simulink model "LoadFlow116BusNetwork_original"  (R2024a)
settings: Solver=FixedStepDiscrete  StartTime=0.0  StopTime=4.5  FixedStep=75e-6  RelTol=1e-3  EnableMultiTasking=on
undefined symbols (not defined in the file or in its folder): D1, D11, Delta
libraries: spsSeriesRLCBranchLib x164, spsLoadFlowBusLib x116, spsDistributedParametersLineLib x79, spsThreePhaseSeriesRLCLoadLib x60, spsThreePhaseTransformerTwoWindingsLib x52, spsThreePhaseParallelRLCLoadLib x44, spsThreePhaseVIMeasurementLib x44, spsSynchronousMachinepuStandardLib x28, spsExcitationSystemLib x28, spsHydraulicTurbineandGovernorLib x28, spsGenericPowerSystemStabilizerLib x28, spsMultiBandPowerSystemStabilizerLib x28
(part 4 of 15)

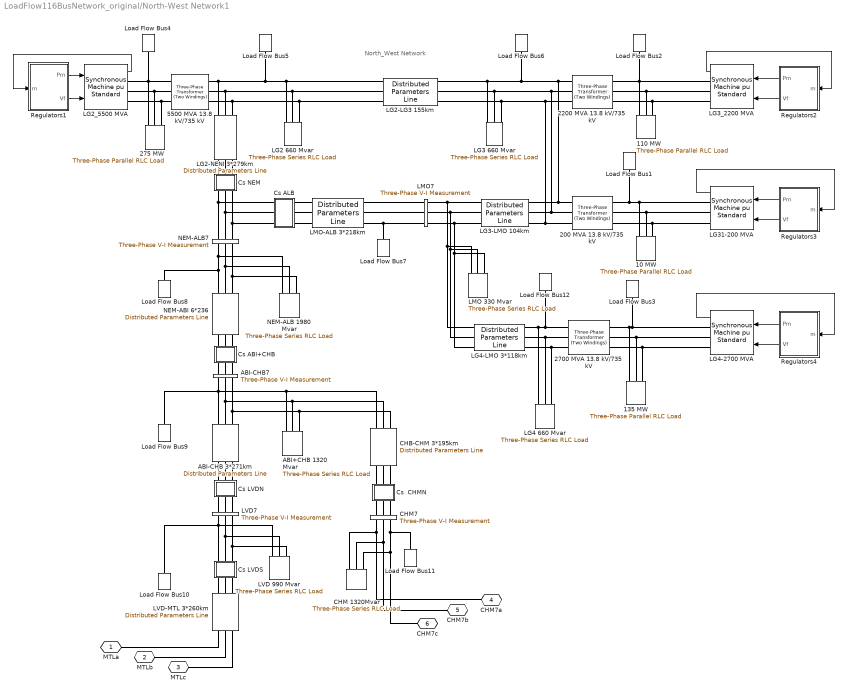
== system LoadFlow116BusNetwork_original/North-West Network1 ==
  note: North_West Network
  10 MW : spsThreePhaseParallelRLCLoadLib/Three-Phase Parallel RLC Load  LConnTagsString=A|B|C  Configuration=Y (grounded)  NominalVoltage=(13800)*1  Vabc=[1e3 1e3 1e3]  Vabcp=[1e3 1e3 1e3]  NominalFrequency=60  UnbalancedPower=off  ActivePower=10000000  InductivePower=0  CapacitivePower=0  Pabc=[10e3 9e3 11e3]  QLabc=[100 90 110]  QCabc=[100 90 110]  Pabcp=[10e3 9e3 11e3]  QLabcp=[100 90 110]  QCabcp=[100 90 110]  Measurements=None  LoadType=constant PQ
  110 MW : spsThreePhaseParallelRLCLoadLib/Three-Phase Parallel RLC Load  LConnTagsString=A|B|C  Configuration=Y (grounded)  NominalVoltage=(13800)*1  Vabc=[1e3 1e3 1e3]  Vabcp=[1e3 1e3 1e3]  NominalFrequency=60  UnbalancedPower=off  ActivePower=110000000  InductivePower=0  CapacitivePower=0  Pabc=[10e3 9e3 11e3]  QLabc=[100 90 110]  QCabc=[100 90 110]  Pabcp=[10e3 9e3 11e3]  QLabcp=[100 90 110]  QCabcp=[100 90 110]  Measurements=None  LoadType=constant PQ
  135 MW : spsThreePhaseParallelRLCLoadLib/Three-Phase Parallel RLC Load  LConnTagsString=A|B|C  Configuration=Y (grounded)  NominalVoltage=(13800)*1  Vabc=[1e3 1e3 1e3]  Vabcp=[1e3 1e3 1e3]  NominalFrequency=60  UnbalancedPower=off  ActivePower=135000000  InductivePower=0  CapacitivePower=0  Pabc=[10e3 9e3 11e3]  QLabc=[100 90 110]  QCabc=[100 90 110]  Pabcp=[10e3 9e3 11e3]  QLabcp=[100 90 110]  QCabcp=[100 90 110]  Measurements=None  LoadType=constant PQ
  200 MVA 13.8 kV/735 kV : spsThreePhaseTransformerTwoWindingsLib/Three-Phase Transformer (Two Windings)  Winding1Connection=Delta (D1)  Winding2Connection=Yg  CoreType=Three single-phase transformers  SetSaturation=off  Hysteresis=off  DataFile='basic_model'  SetInitialFlux=off  Measurements=None  UNITS=pu  NominalPower=[ 200e6 60 ]  Winding1="[ 13.8e3 0.002  0.0]"  Winding2=[ 735e3 0.002 0.12]  Rm=500  Lm=500  L0=0.5  Saturation="[ 0,0  ;  0.005,1.2  ;  1.0,1.4 ]"  InitialFluxes=[ 0.8 , -0.8 , 0.7 ]  BreakLoop=off  DiscreteSolver=Trapezoidal iterative  DataType=off  TransfoNumber=0
  2200 MVA 13.8 kV/735 kV : spsThreePhaseTransformerTwoWindingsLib/Three-Phase Transformer (Two Windings)  Winding1Connection=Delta (D1)  Winding2Connection=Yg  CoreType=Three single-phase transformers  SetSaturation=off  Hysteresis=off  DataFile='basic_model'  SetInitialFlux=off  Measurements=None  UNITS=pu  NominalPower=[ 2200e6 60 ]  Winding1="[ 13.8e3 0.002  0.0]"  Winding2=[ 735e3 0.002 0.12]  Rm=500  Lm=500  L0=0.5  Saturation="[ 0,0  ;  0.005,1.2  ;  1.0,1.4 ]"  InitialFluxes=[ 0.8 , -0.8 , 0.7 ]  BreakLoop=off  DiscreteSolver=Trapezoidal iterative  DataType=off  TransfoNumber=0
  2700 MVA 13.8 kV/735 kV : spsThreePhaseTransformerTwoWindingsLib/Three-Phase Transformer (Two Windings)  Winding1Connection=Delta (D1)  Winding2Connection=Yg  CoreType=Three single-phase transformers  SetSaturation=off  Hysteresis=off  DataFile='basic_model'  SetInitialFlux=off  Measurements=None  UNITS=pu  NominalPower=[ 2700e6 60 ]  Winding1="[ 13.8e3 0.002  0.0]"  Winding2=[ 735e3 0.002 0.12]  Rm=500  Lm=500  L0=0.5  Saturation="[ 0,0  ;  0.005,1.2  ;  1.0,1.4 ]"  InitialFluxes=[ 0.8 , -0.8 , 0.7 ]  BreakLoop=off  DiscreteSolver=Trapezoidal iterative  DataType=off  TransfoNumber=0
  275 MW : spsThreePhaseParallelRLCLoadLib/Three-Phase Parallel RLC Load  LConnTagsString=A|B|C  Configuration=Y (grounded)  NominalVoltage=(13800)*1  Vabc=[1e3 1e3 1e3]  Vabcp=[1e3 1e3 1e3]  NominalFrequency=60  UnbalancedPower=off  ActivePower=275000000  InductivePower=0  CapacitivePower=0  Pabc=[10e3 9e3 11e3]  QLabc=[100 90 110]  QCabc=[100 90 110]  Pabcp=[10e3 9e3 11e3]  QLabcp=[100 90 110]  QCabcp=[100 90 110]  Measurements=None  LoadType=constant PQ
  5500 MVA 13.8 kV/735 kV : spsThreePhaseTransformerTwoWindingsLib/Three-Phase Transformer (Two Windings)  Winding1Connection=Delta (D1)  Winding2Connection=Yg  CoreType=Three single-phase transformers  SetSaturation=off  Hysteresis=off  DataFile='basic_model'  SetInitialFlux=off  Measurements=None  UNITS=pu  NominalPower=[ 5500e6 60 ]  Winding1="[ 13.8e3 0.002  0.0]"  Winding2=[ 735e3 0.002 0.12]  Rm=500  Lm=500  L0=0.5  Saturation="[ 0,0  ;  0.005,1.2  ;  1.0,1.4 ]"  InitialFluxes=[ 0.8 , -0.8 , 0.7 ]  BreakLoop=off  DiscreteSolver=Trapezoidal iterative  DataType=off  TransfoNumber=0
  ABI+CHB 1320 Mvar : spsThreePhaseSeriesRLCLoadLib/Three-Phase Series RLC Load  LConnTagsString=A|B|C  Configuration=Y (grounded)  NominalVoltage=735e3  Vabc=[1e3 1e3 1e3]  Vabcp=[1e3 1e3 1e3]  NominalFrequency=60  UnbalancedPower=off  ActivePower=4400000  InductivePower=1320e6  CapacitivePower=0  Pabc=[10e3 9e3 11e3]  QLabc=[100 90 110]  QCabc=[100 90 110]  Pabcp=[10e3 9e3 11e3]  QLabcp=[100 90 110]  QCabcp=[100 90 110]  Measurements=None  LoadType=constant Z
  ABI-CHB 3*271km : spsDistributedParametersLineLib/Distributed Parameters Line  Phases=3  Length=271  Frequency=60  Resistance="[0.01273  0.3864]/3"  Inductance="[0.9337e-3  4.1264e-3]/3"  Capacitance=[12.74e-9 7.751e-9]*3  x1=[-0.001575 8.53864444420272e-09 -6095.79039975099 -646119.037388367;-0.0015 8.97910610131053e-09 12172.7797949347 -646033.10373521;-0.001425 9.41238999838588e-09 30431.6192557021 -645430.741103565;-0.00135 9.83814977491093e-09 48666.1321456558 -644312.431012903;-0.001275 1.02560450850346e-08 66861.7420741891 -642679.0674232;-0.0012 1.06657418696401e-08 85003.9037491273 -640531.956020319;-0.001125 1.10669126233864e-08 103078.114604012 -637872.813172263;-0.00105 1.14592366565109e-08 121069.92639123 -634703.764557137;-0.000975 1.18424003511844e-08 138964.956731723 -631027.343463919;-0.0009 1.2216097412212e-08 156748.900612039 -626846.488767377;-0.000825 1.25800291118808e-08 174407.541819545 -622164.542578787;-0.00075 1.29339045287585e-08 191926.764306646 -616985.247574297;-0.000675 1.32774407802513e-08 209292.563474937 -611312.744003087;-0.0006 1.36103632487359e-08 226491.057370271 -605151.566377719;-0.000525 1.39324058010851e-08 243508.497779772 -598506.639849319;-0.00045 1.42433110014099e-08 260331.281221952 -591383.276270481;-0.000375 1.45428303168501e-08 276945.959821126 -583787.169949061;-0.0003 1.48307243162478e-08 293339.252057435 -575724.393096226;-0.000225 1.51067628615447e-08 309498.053383889 -567201.390972429;-0.00015 1.53707252917514e-08 325409.446701948 -558224.976735161;-7.5e-05 1.56224005993398e-08 341060.712687245 -548802.325992619]  x2=[-0.001575 1.88534480665931e-08 -248614.692980958 -602078.188381427;-0.0015 1.97916287683191e-08 -231494.235349789 -608866.016701703;-0.001425 2.07139883448297e-08 -214188.724768862 -615167.126844189;-0.00135 2.16197894759921e-08 -196711.994998552 -620976.481797849;-0.001275 2.25083080782413e-08 -179078.016669235 -626289.437653218;-0.0012 2.33788338834014e-08 -161300.886113378 -631101.747314677;-0.001125 2.42306710064632e-08 -143394.814097148 -635409.563895514;-0.00105 2.50631385018642e-08 -125374.114460544 -639209.443793065;-0.000975 2.58755709078257e-08 -107253.192675128 -642498.349441479;-0.0009 2.6667318778313e-08 -89046.5343285159 -645273.651739905;-0.000825 2.74377492021925e-08 -70768.6935448196 -647533.132154148;-0.00075 2.81862463091715e-08 -52434.2813503008 -649274.984490136;-0.000675 2.89122117621149e-08 -34057.953993542 -650497.816337763;-0.0006 2.96150652353474e-08 -15654.401229465 -651200.65018396;-0.000525 3.02942448785564e-08 2761.66542343446 -651382.924194104;-0.00045 3.0949207765927e-08 21175.5244432494 -651044.49266114;-0.000375 3.15794303301483e-08 39572.4560728207 -650185.626122058;-0.0003 3.21844087809452e-08 57937.7540864864 -648807.011141627;-0.000225 3.27636595078005e-08 76256.7375460126 -646909.74976357;-0.00015 3.33167194665461e-08 94514.7625363118 -644495.358629602;-7.5e-05 3.3843146549513e-08 112697.233871564 -641565.767767057]  x3=[-0.001575 -8.90212723717372e-11 -202.312158707681 698.106439471244;-0.0015 -8.43577927577515e-11 -221.966976544963 692.108516415909;-0.001425 -7.96268788149527e-11 -241.444357377404 685.557332402166;-0.00135 -7.48323123635614e-11 -260.72873128478 678.458124346279;-0.001275 -6.99779261066394e-11 -279.804682633651 670.816567246548;-0.0012 -6.5067600566286e-11 -298.656962400379 662.638769646797;-0.001125 -6.01052609816075e-11 -317.270500360969 653.931268753304;-0.00105 -5.50948741709416e-11 -335.630417137972 644.701025209054;-0.000975 -5.00404453608434e-11 -353.722036094833 634.955417529507;-0.0009 -4.49460149843682e-11 -371.530895068167 624.702236204332;-0.000825 -3.98156554512116e-11 -389.042757928598 613.949677469799;-0.00075 -3.46534678922872e-11 -406.243625960894 602.706336756842;-0.000675 -2.94635788813456e-11 -423.119749054334 590.981201819998;-0.0006 -2.42501371362541e-11 -439.657636694328 578.783645552735;-0.000525 -1.90173102025754e-11 -455.844068746536 566.123418494903;-0.00045 -1.37692811220954e-11 -471.666106024837 553.010641038306;-0.000375 -8.51024508896343e-12 -487.111100634715 539.455795336609;-0.0003 -3.24440609611847e-12 -502.166706083795 525.46971692607;-0.000225 2.02402642531864e-12 -516.82088715144 511.063586063777;-0.00015 7.290840971e-12 -531.061929509521 496.248918790319;-7.5e-05 1.25518273299627e-11 -544.878449086672 481.037557724044]  x4=[-0.001575 1.31429208848847e-10 -5039.99478840298 -13897.9312159916;-0.0015 1.32758724317523e-10 -4645.07840312877 -14034.8602322785;-0.001425 1.33982114493257e-10 -4246.44881325117 -14160.5699960362;-0.00135 1.3509840141666e-10 -3844.42467716511 -14274.9600168031;-0.001275 1.36106692745046e-10 -3439.32736681379 -14377.9388529468;-0.0012 1.37006182465753e-10 -3031.48071078892 -14469.4241847613;-0.001125 1.37796151540462e-10 -2621.21073546704 -14549.3428802721;-0.00105 1.38475968479981e-10 -2208.84540438911 -14617.6310536968;-0.000975 1.39045089849051e-10 -1794.71435609138 -14674.2341165144;-0.0009 1.39503060700757e-10 -1379.14864059743 -14719.1068211026;-0.000825 1.39849514940207e-10 -962.480454781879 -14752.213296908;-0.00075 1.40084175617183e-10 -545.042876817216 -14773.5270791201;-0.000675 1.4020685514753e-10 -127.169599916261 -14783.0311298278;-0.0006 1.4021745546311e-10 290.805334417106 -14780.7178516383;-0.000525 1.40115968090191e-10 708.547803415612 -14766.5890937507;-0.00045 1.39902474156227e-10 1125.72387014121 -14740.656150478;-0.000375 1.39577144325002e-10 1542.00005042917 -14702.9397522182;-0.0003 1.39140238660206e-10 1957.04357947021 -14653.470048883;-0.000225 1.38592106417542e-10 2370.5226778176 -14592.2865857963;-0.00015 1.37933185765538e-10 2782.10681660655 -14519.4382720824;-7.5e-05 1.37164003435281e-10 3191.46698177396 -14434.9833415687]  x5=0.00153261764655846  V1=ones(3,3)  V2=ones(3,3)  I1=ones(3,3)  I2=ones(3,3)  nHarmo=1  Measurements=None  Decoupling=off  VsMag0=[ 1 1 1]  VrMag0=[ 1 1 1]  VsAngle0=[0 -120 120]  VrAngle0=[0 -120 120]  IsMag0=[ 1 1 1]  IrMag0=[ 1 1 1]  IsAngle0=[0 -120 120]  IrAngle0=[0 -120 120]
      settings: AttributesFormatString=\n  LibrarySourceBlock=sps_lib/Power Grid Elements/Distributed Parameters Line
  ABI-CHB7 : spsThreePhaseVIMeasurementLib/Three-Phase V-I Measurement  VoltageMeasurement=no  SetLabelV=on  LabelV=Vabc_ABI7  Vpu=on  VpuLL=off  CurrentMeasurement=no  SetLabelI=off  LabelI=A1  Ipu=off  Pbase=100e6  Vbase=500e3  OutputType=Magnitude  PhasorSimulation=off  PSBequivalent=0
  CHB-CHM 3*195km : spsDistributedParametersLineLib/Distributed Parameters Line  Phases=3  Length=195  Frequency=60  Resistance="[0.01273  0.3864]/3"  Inductance="[0.9337e-3  4.1264e-3]/3"  Capacitance=[12.74e-9 7.751e-9]*3  x1=[-0.001125 1.10669126233864e-08 0 0;-0.00105 1.14592366565109e-08 0 0;-0.000975 1.18424003511844e-08 0 0;-0.0009 1.2216097412212e-08 0 0;-0.000825 1.25800291118808e-08 0 0;-0.00075 1.29339045287585e-08 0 0;-0.000675 1.32774407802513e-08 209292.563474937 -611312.744003087;-0.0006 1.36103632487359e-08 226491.057370271 -605151.566377719;-0.000525 1.39324058010851e-08 243508.497779772 -598506.639849319;-0.00045 1.42433110014099e-08 260331.281221952 -591383.276270481;-0.000375 1.45428303168501e-08 276945.959821126 -583787.169949061;-0.0003 1.48307243162478e-08 293339.252057435 -575724.393096226;-0.000225 1.51067628615447e-08 309498.053383889 -567201.390972429;-0.00015 1.53707252917514e-08 325409.446701948 -558224.976735161;-7.5e-05 1.56224005993398e-08 341060.712687245 -548802.325992619]  x2=[-0.001125 8.59552162662043e-09 0 0;-0.00105 8.86565649966125e-09 0 0;-0.000975 9.12870430254534e-09 0 0;-0.0009 9.38445475888383e-09 0 0;-0.000825 9.63270342567504e-09 0 0;-0.00075 9.87325185673308e-09 0 0;-0.000675 1.01059077613227e-08 111004.534524816 -639558.940614591;-0.0006 1.03304851578734e-08 129040.856793898 -636165.151877435;-0.000525 1.05468045226507e-08 146974.025776451 -632262.822451521;-0.00045 1.07546929332641e-08 164789.705971576 -627855.071799286;-0.000375 1.09539842068989e-08 182473.655797114 -622945.423409158;-0.0003 1.11445190331604e-08 200011.738974149 -617537.801978942;-0.000225 1.13261451014236e-08 217389.93582733 -611636.530278469;-0.00015 1.14987172225885e-08 234594.354491989 -605246.325694044;-7.5e-05 1.1662097445142e-08 251611.24201908 -598372.296457439]  x3=[-0.001125 6.30139306376083e-11 0 0;-0.00105 6.39237031354486e-11 0 0;-0.000975 6.47823760030679e-11 0 0;-0.0009 6.55892628305139e-11 0 0;-0.000825 6.63437186048026e-11 0 0;-0.00075 6.70451402255315e-11 0 0;-0.000675 6.76929669869892e-11 49.2476883451471 -2749.35029594662;-0.0006 6.82866810263746e-11 126.95444951433 -2746.85863033986;-0.000525 6.88258077377687e-11 204.55972523904 -2742.17116797236;-0.00045 6.93099161515275e-11 282.001479049262 -2735.2916559298;-0.000375 6.9738619278792e-11 359.2178051919 -2726.22559358886;-0.0003 7.01115744208418e-11 436.146978117284 -2714.98022822106;-0.000225 7.04284834430425e-11 512.727501821634 -2701.5645491994;-0.00015 7.06890930131708e-11 588.898159006021 -2685.98928081244;-7.5e-05 7.08931948039238e-11 664.598060012543 -2668.26687369142]  x4=[-0.001125 -1.1064985641538e-11 0 0;-0.00105 -8.88435086725677e-12 0 0;-0.000975 -6.69661407882735e-12 0 0;-0.0009 -4.50352411956495e-12 0 0;-0.000825 -2.30683411202761e-12 0 0;-0.00075 -1.08300056596849e-13 0 0;-0.000675 2.09032057224212e-12 1717.04187839405 -11467.1483442372;-0.0006 4.2872702307986e-12 2040.53742261431 -11414.0235556945;-0.000525 6.48079271113001e-12 2362.4017924402 -11351.7745713617;-0.00045 8.66913454492761e-12 2682.37769441917 -11280.4511521246;-0.000375 1.08505464052122e-11 3000.20934471098 -11200.1103128332;-0.0003 1.30232845047194e-11 3315.64267355737 -11110.8162767252;-0.000225 1.51856119898564e-11 3628.42552838155 -11012.6404240867;-0.00015 1.73358003291164e-11 3938.30787535512 -10905.6612351922;-7.5e-05 1.947213069484e-11 4245.04199927126 -10789.9642275686]  x5=0.0011028060556417  V1=ones(3,3)  V2=ones(3,3)  I1=ones(3,3)  I2=ones(3,3)  nHarmo=1  Measurements=None  Decoupling=off  VsMag0=[ 1 1 1]  VrMag0=[ 1 1 1]  VsAngle0=[0 -120 120]  VrAngle0=[0 -120 120]  IsMag0=[ 1 1 1]  IrMag0=[ 1 1 1]  IsAngle0=[0 -120 120]  IrAngle0=[0 -120 120]
      settings: AttributesFormatString=\n  LibrarySourceBlock=sps_lib/Power Grid Elements/Distributed Parameters Line
  CHM 1320Mvar : spsThreePhaseSeriesRLCLoadLib/Three-Phase Series RLC Load  LConnTagsString=A|B|C  Configuration=Y (grounded)  NominalVoltage=735e3  Vabc=[1e3 1e3 1e3]  Vabcp=[1e3 1e3 1e3]  NominalFrequency=60  UnbalancedPower=off  ActivePower=4400000  InductivePower=1320e6  CapacitivePower=0  Pabc=[10e3 9e3 11e3]  QLabc=[100 90 110]  QCabc=[100 90 110]  Pabcp=[10e3 9e3 11e3]  QLabcp=[100 90 110]  QCabcp=[100 90 110]  Measurements=None  LoadType=constant Z
  CHM7 : spsThreePhaseVIMeasurementLib/Three-Phase V-I Measurement  VoltageMeasurement=no  SetLabelV=on  LabelV=Vabc_CHM7  Vpu=on  VpuLL=off  CurrentMeasurement=no  SetLabelI=off  LabelI=A1  Ipu=off  Pbase=100e6  Vbase=735e3  OutputType=Magnitude  PhasorSimulation=off  PSBequivalent=0
  "Cs  CHMN " : Subsystem  mask{Xc=25/3}
      mask prompts: Xc "Condensator Reactance at  60Hz  (ohm):"
      mask help: Series Compensation
      mask init:
      | Cs=1/Xc/(2*pi*60);
      mask Display: disp('Cs')
  "Cs ABI+CHB " : Subsystem  mask{Xc=25/6}
      mask prompts: Xc "Condensator Reactance at  60Hz  (ohm):"
      mask help: Series Compensation
      mask init:
      | Cs=1/Xc/(2*pi*60);
      mask Display: disp('Cs')
  Cs ALB : Subsystem  mask{Xc=16/3}
      mask prompts: Xc "Reactance @ 60Hz du condensateur (ohm):"
      mask init:
      | Cs=1/Xc/(2*pi*60);
      mask Display: disp('Cs')
  "Cs LVDN " : Subsystem  mask{Xc=34/3}
      mask prompts: Xc "Condensator Reactance at  60Hz  (ohm):"
      mask help: Series Compensation
      mask init:
      | Cs=1/Xc/(2*pi*60);
      mask Display: disp('Cs')
  "Cs LVDS " : Subsystem  mask{Xc=34/3}
      mask prompts: Xc "Condensator Reactance at  60Hz  (ohm):"
      mask help: Series Compensation
      mask init:
      | Cs=1/Xc/(2*pi*60);
      mask Display: disp('Cs')
  "Cs NEM " : Subsystem  mask{Xc=16/3}
      mask prompts: Xc "Condensator Reactance at  60Hz  (ohm):"
      mask help: Series Compensation
      mask init:
      | Cs=1/Xc/(2*pi*60);
      mask Display: disp('Cs')
  LG2 660 Mvar : spsThreePhaseSeriesRLCLoadLib/Three-Phase Series RLC Load  LConnTagsString=A|B|C  Configuration=Y (grounded)  NominalVoltage=735e3  Vabc=[1e3 1e3 1e3]  Vabcp=[1e3 1e3 1e3]  NominalFrequency=60  UnbalancedPower=off  ActivePower=2200000  InductivePower=660e6  CapacitivePower=0  Pabc=[10e3 9e3 11e3]  QLabc=[100 90 110]  QCabc=[100 90 110]  Pabcp=[10e3 9e3 11e3]  QLabcp=[100 90 110]  QCabcp=[100 90 110]  Measurements=None  LoadType=constant Z
  LG2-LG3 155km : spsDistributedParametersLineLib/Distributed Parameters Line  Phases=3  Length=155  Frequency=60  Resistance="[0.01273  0.3864]"  Inductance="[0.9337e-3  4.1264e-3]"  Capacitance=[12.74e-9 7.751e-9]  x1=[-0.0009 -9.28273050085322e-10 431553.276717529 -473538.091690319;-0.000825 -8.70852358492143e-10 444767.945318795 -461148.506915131;-0.00075 -8.12735520848074e-10 457627.073229751 -448390.287079324;-0.000675 -7.53968994863909e-10 470120.381060296 -435273.630908626;-0.0006 -6.94599757601362e-10 482237.881851304 -421809.023657291;-0.000525 -6.34675267920321e-10 493969.889058048 -408007.228726338;-0.00045 -5.74243428540962e-10 505307.024293471 -393879.279059461;-0.000375 -5.13352547751047e-10 516240.224825131 -379436.468323459;-0.0003 -4.52051300789016e-10 526760.750819806 -364690.341880252;-0.000225 -3.90388690933752e-10 536860.192329986 -349652.687557696;-0.00015 -3.28414010332102e-10 546530.476016653 -334335.526226571;-7.5e-05 -2.66176800595496e-10 555763.871602989 -318751.102191286]  x2=[-0.0009 -4.73016797850604e-10 434484.753049023 -467489.581126984;-0.000825 -4.96742942646812e-10 447527.255751984 -455019.542461771;-0.00075 -5.2007199873509e-10 460212.012014093 -442185.768136346;-0.000675 -5.42985317224948e-10 472528.881835278 -428998.517273542;-0.0006 -5.6546458156017e-10 484468.019298258 -415468.331559927;-0.000525 -5.87491822160791e-10 496019.88043922 -401606.026818942;-0.00045 -6.09049430787703e-10 507175.230877118 -387422.684364896;-0.000375 -6.30120174618412e-10 517925.153195494 -372929.642144734;-0.0003 -6.50687210022693e-10 528261.054070926 -358138.485674657;-0.000225 -6.70734096027131e-10 538174.671142399 -343061.038778834;-0.00015 -6.90244807457779e-10 547658.079616109 -327709.354137622;-7.5e-05 -7.09203747750446e-10 556703.698600424 -312095.703652832]  x3=[-0.0009 8.7944193226646e-12 1522.16056329666 -1950.05893522532;-0.000825 8.80014406364708e-12 1576.68135164224 -1906.24695426432;-0.00075 8.79883410411181e-12 1629.94176503934 -1860.91114865463;-0.000675 8.79049049122039e-12 1681.89922792843 -1814.0877591456;-0.0006 8.7751198947293e-12 1732.51220630862 -1765.81421563838;-0.000525 8.7527346016582e-12 1781.74024093942 -1716.12910726505;-0.00045 8.72335250646786e-12 1829.54397968315 -1665.07215154102;-0.000375 8.68699709675562e-12 1875.88520896249 -1612.68416261551;-0.0003 8.64369743447975e-12 1920.72688430778 -1559.0070186453;-0.000225 8.59348813272776e-12 1964.03315996987 -1504.08362831799;-0.00015 8.53640932804725e-12 2005.76941757459 -1447.95789655146;-7.5e-05 8.47250664836133e-12 2045.90229379621 -1390.67468939692]  x4=[-0.0009 -1.19841358644897e-11 1309.19110331829 -1829.24101140887;-0.000825 -1.1964801318714e-11 1360.38131280582 -1791.49811725853;-0.00075 -1.19359022938317e-11 1410.48405428643 -1752.3231269241;-0.000675 -1.18974618912811e-11 1459.45927639517 -1711.74735629344;-0.0006 -1.18495108397319e-11 1507.26782908884 -1669.80324101677;-0.000525 -1.1792087470521e-11 1553.8714949419 -1626.52431057809;-0.00045 -1.17252376870111e-11 1599.23301969694 -1581.94516149218;-0.000375 -1.16490149278965e-11 1643.31614204512 -1536.10142964875;-0.0003 -1.15634801244843e-11 1686.08562261293 -1489.02976182559;-0.000225 -1.14687016519879e-11 1727.50727213199 -1440.76778639376;-0.00015 -1.13647552748678e-11 1767.54797876946 -1391.35408323796;-7.5e-05 -1.12517240862676e-11 1806.1757345971 -1340.82815291646]  x5=0.000876589428843401  V1=ones(3,3)  V2=ones(3,3)  I1=ones(3,3)  I2=ones(3,3)  nHarmo=1  Measurements=None  Decoupling=off  VsMag0=[ 1 1 1]  VrMag0=[ 1 1 1]  VsAngle0=[0 -120 120]  VrAngle0=[0 -120 120]  IsMag0=[ 1 1 1]  IrMag0=[ 1 1 1]  IsAngle0=[0 -120 120]  IrAngle0=[0 -120 120]
      settings: AttributesFormatString=\n  LibrarySourceBlock=sps_lib/Power Grid Elements/Distributed Parameters Line
  LG2-NENI 3*279km : spsDistributedParametersLineLib/Distributed Parameters Line  Phases=3  Length=279  Frequency=60  Resistance="[0.01273  0.3864]/3"  Inductance="[0.9337e-3  4.1264e-3]/3"  Capacitance=[12.74e-9 7.751e-9]*3  x1=[-0.00165 -1.45441548682992e-09 282305.297313422 -575135.752528875;-0.001575 -1.40637124143826e-09 298451.827359304 -566924.896508615;-0.0015 -1.3572027643944e-09 314359.779580861 -558260.849400328;-0.001425 -1.30694936022658e-09 330016.437404487 -549150.537110708;-0.00135 -1.25565120073718e-09 345409.285137473 -539601.242284006;-0.001275 -1.20334929289003e-09 360526.017972859 -529620.598480399;-0.0012 -1.15008544603e-09 375354.551825711 -519216.584073833;-0.001125 -1.09590223846132e-09 389883.03299295 -508397.515874239;-0.00105 -1.04084298341107e-09 404099.847629026 -497172.042479198;-0.000975 -9.84951694405317e-10 417993.631029841 -485549.137360386;-0.0009 -9.28273050085322e-10 431553.276717529 -473538.091690319;-0.000825 -8.70852358492143e-10 444767.945318795 -461148.506915131;-0.00075 -8.12735520848074e-10 457627.073229751 -448390.287079324;-0.000675 -7.53968994863909e-10 470120.381060296 -435273.630908626;-0.0006 -6.94599757601362e-10 482237.881851304 -421809.023657291;-0.000525 -6.34675267920321e-10 493969.889058048 -408007.228726338;-0.00045 -5.74243428540962e-10 505307.024293471 -393879.279059461;-0.000375 -5.13352547751047e-10 516240.224825131 -379436.468323459;-0.0003 -4.52051300789016e-10 526760.750819806 -364690.341880252;-0.000225 -3.90388690933752e-10 536860.192329986 -349652.687557696;-0.00015 -3.28414010332102e-10 546530.476016653 -334335.526226571;-7.5e-05 -2.66176800595496e-10 555763.871602989 -318751.102191286]  x2=[-0.00165 4.87150453497474e-09 59028.0607460847 -635612.648559132;-0.001575 5.14344828048769e-09 76973.5739080496 -633689.821780515;-0.0015 5.41128043214263e-09 94857.5555727677 -631260.433054146;-0.001425 5.67478688901547e-09 112665.70955893 -628326.424396202;-0.00135 5.93375700807639e-09 130383.800300714 -624890.141208313;-0.001275 6.18798377257458e-09 147997.664227477 -620954.330402681;-0.0012 6.4372639575243e-09 165493.221085897 -616522.138206246;-0.001125 6.68139829215981e-09 182856.485195511 -611597.107645633;-0.00105 6.9201916192294e-09 200073.576628659 -606183.175714918;-0.000975 7.15345305100105e-09 217130.732305878 -600284.67022845;-0.0009 7.38099612185524e-09 234014.316997903 -593906.306361265;-0.000825 7.60263893734264e-09 250710.834225459 -587053.182879846;-0.00075 7.81820431958781e-09 267206.93704814 -579730.778066247;-0.000675 8.02751994892244e-09 283489.438733748 -571944.945338841;-0.0006 8.23041850163507e-09 299545.323299565 -563701.908573182;-0.000525 8.42673778372712e-09 315361.755917135 -555008.257126738;-0.00045 8.61632086056827e-09 330926.093172221 -545870.940571458;-0.000375 8.79901618234761e-09 346225.893171763 -536297.263138391;-0.0003 8.97467770522025e-09 361248.925489739 -526294.877878794;-0.000225 9.14316500805251e-09 375983.180943971 -515871.780546403;-0.00015 9.30434340467244e-09 390416.881196093 -505036.303205745;-7.5e-05 9.45808405153591e-09 404538.488166965 -493797.10757162]  x3=[-0.00165 -4.70582752222005e-11 -180.946605755205 -28.0430826428717;-0.001575 -4.53728751740235e-11 -180.08124143958 -33.1461710872375;-0.0015 -4.36512047436605e-11 -179.071922934883 -38.2227629895896;-0.001425 -4.18946402081113e-11 -177.919457074885 -43.2688002000357;-0.00135 -4.01045857381892e-11 -176.624765123161 -48.2802489936368;-0.001275 -3.82824722760488e-11 -175.188882036646 -53.2531032949049;-0.0012 -3.64297563913123e-11 -173.612955638311 -58.1833878801989;-0.001125 -3.45479191167106e-11 -171.898245699606 -63.0671615554571;-0.00105 -3.26384647641679e-11 -170.04612293342 -67.9005203067278;-0.000975 -3.0702919722278e-11 -168.058067898354 -72.6796004209782;-0.0009 -2.87428312361325e-11 -165.935669815185 -77.4005815746872;-0.000825 -2.67597661704769e-11 -163.680625296466 -82.0596898877539;-0.00075 -2.47553097571828e-11 -161.294736990283 -86.6532009402798;-0.000675 -2.27310643280377e-11 -158.779912139242 -91.1774427498124;-0.0006 -2.06886480338658e-11 -156.138161055851 -95.6287987066725;-0.000525 -1.86296935510025e-11 -153.371595515506 -100.003710465016;-0.00045 -1.65558467761584e-11 -150.48242706837 -104.298680787322;-0.000375 -1.44687655107144e-11 -147.472965271494 -108.51027634003;-0.0003 -1.23701181355006e-11 -144.345615842592 -112.635130438095;-0.000225 -1.02615822771185e-11 -141.102878736948 -116.669945736263;-0.00015 -8.14484346687156e-12 -137.747346148987 -120.611496864919;-7.5e-05 -6.02159379337746e-12 -134.28170044012 -124.456633008399]  x4=[-0.00165 4.85330925004575e-11 1481.48089108514 -13945.3845775473;-0.001575 4.8116399182976e-11 1875.13150496029 -13897.9289700678;-0.0015 4.76612423521933e-11 2267.28316740084 -13839.3635708151;-0.001425 4.71679858535157e-11 2657.62239836797 -13769.7351960732;-0.00135 4.66370239886411e-11 3045.83716665283 -13689.0995056996;-0.001275 4.60687812003605e-11 3431.61713930954 -13597.5209586313;-0.0012 4.54637117332642e-11 3814.65392973059 -13495.0727613578;-0.001125 4.48222992706266e-11 4194.64134416638 -13381.8368094004;-0.00105 4.41450565477561e-11 4571.2756264918 -13257.9036218466;-0.000975 4.34325249421234e-11 4944.25570102427 -13123.3722689901;-0.0009 4.26852740405918e-11 5313.28341319899 -12978.3502931362;-0.000825 4.19039011840989e-11 5678.06376790915 -12822.9536226333;-0.00075 4.10890309901505e-11 6038.30516532055 -12657.3064792023;-0.000675 4.02413148535119e-11 6393.71963397195 -12481.5412786351;-0.0006 3.93614304254921e-11 6744.02306097514 -12295.7985249437;-0.000525 3.84500810722403e-11 7088.93541913041 -12100.2266980435;-0.00045 3.75079953124852e-11 7428.18099077597 -11894.9821350606;-0.000375 3.6535926235169e-11 7761.48858819248 -11680.2289053583;-0.0003 3.55346508974388e-11 8088.59177038635 -11456.1386793825;-0.000225 3.45049697034795e-11 8409.22905607858 -11222.8905914312;-0.00015 3.34477057646831e-11 8723.1441327289 -10980.671096457;-7.5e-05 3.23637042416654e-11 9030.0860614281 -10729.6738210183]  x5=0.00157786097191812  V1=ones(3,3)  V2=ones(3,3)  I1=ones(3,3)  I2=ones(3,3)  nHarmo=1  Measurements=None  Decoupling=off  VsMag0=[ 1 1 1]  VrMag0=[ 1 1 1]  VsAngle0=[0 -120 120]  VrAngle0=[0 -120 120]  IsMag0=[ 1 1 1]  IrMag0=[ 1 1 1]  IsAngle0=[0 -120 120]  IrAngle0=[0 -120 120]
      settings: AttributesFormatString=\n  LibrarySourceBlock=sps_lib/Power Grid Elements/Distributed Parameters Line
  LG2_5500 MVA : spsSynchronousMachinepuStandardLib/Synchronous Machine pu Standard  PresetModel=No  MechanicalLoad=Mechanical power Pm  ShowDetailedParameters=on  RotorType=Salient-pole  Units=per unit standard parameters  MeasurementBus=off  NominalParameters="[5500E6  13800   60 ]"  Reactances1=[ 31 32 33 34 35 36 37 ]  Reactances2=[ 1.305, 0.296, 0.252, 0.474, 0.243, 0.18 ]  dAxisTimeConstants=Short-circuit  qAxisTimeConstants=Open-circuit  TimeConstants1=[]  TimeConstants2=[]  TimeConstants3=[]  TimeConstants4=[]  TimeConstants5=[ 1.01, 0.053, 0.1 ]  TimeConstants6=[]  TimeConstants7=[]  TimeConstants8=[]  StatorResistance=2.8544e-3  Mechanical="[ 4.1  0  32]"  PolePairs=32  InitialConditions=[0 -65.2434 0.985682 0.985682 0.985682 -1.22427 -121.224 118.776 1.47412]  SetSaturation=off  Saturation=[0.6404,0.7127,0.8441,0.9214,0.9956,1.082,1.19,1.316,1.457;0.7,0.7698,0.8872,0.9466,0.9969,1.046,1.1,1.151,1.201]  LoadFlowParameters=[2 4000000000 0 0 0]  TsPowergui=0  TsBlock=-1  IterativeModel=Trapezoidal non iterative  IterativeDiscreteModel=Trapezoidal non iterative  BusType=swing  Pref=0  Qref=0  Qmin=-Inf  Qmax=Inf  PLF=0  QLF=0
  LG3 660 Mvar : spsThreePhaseSeriesRLCLoadLib/Three-Phase Series RLC Load  LConnTagsString=A|B|C  Configuration=Y (grounded)  NominalVoltage=735e3  Vabc=[1e3 1e3 1e3]  Vabcp=[1e3 1e3 1e3]  NominalFrequency=60  UnbalancedPower=off  ActivePower=2200000  InductivePower=660e6  CapacitivePower=0  Pabc=[10e3 9e3 11e3]  QLabc=[100 90 110]  QCabc=[100 90 110]  Pabcp=[10e3 9e3 11e3]  QLabcp=[100 90 110]  QCabcp=[100 90 110]  Measurements=None  LoadType=constant Z
  LG3-LMO 104km : spsDistributedParametersLineLib/Distributed Parameters Line  Phases=3  Length=104  Frequency=60  Resistance="[0.01273  0.3864]"  Inductance="[0.9337e-3  4.1264e-3]"  Capacitance=[12.74e-9 7.751e-9]  x1=[-0.0006 -5.6546458156017e-10 0 0;-0.000525 -5.87491822160791e-10 0 0;-0.00045 -6.09049430787703e-10 0 0;-0.000375 -6.30120174618412e-10 517925.153195494 -372929.642144734;-0.0003 -6.50687210022693e-10 528261.054070926 -358138.485674657;-0.000225 -6.70734096027131e-10 538174.671142399 -343061.038778834;-0.00015 -6.90244807457779e-10 547658.079616109 -327709.354137622;-7.5e-05 -7.09203747750446e-10 556703.698600424 -312095.703652832]  x2=[-0.0006 2.62559334955073e-09 0 0;-0.000525 2.68721757878452e-09 0 0;-0.00045 2.74669368740163e-09 0 0;-0.000375 2.80397413111085e-09 463443.99687782 -442193.458727678;-0.0003 2.85901312080191e-09 475759.806920902 -428914.853919972;-0.000225 2.91176665914857e-09 487695.3018537 -415293.38114066;-0.00015 2.96219257577943e-09 499240.940624185 -401339.929186666;-7.5e-05 3.01025056098827e-09 510387.493825377 -387065.652233986]  x3=[-0.0006 -1.23301013005406e-11 0 0;-0.000525 -1.17759417137608e-11 0 0;-0.00045 -1.12123686193529e-11 0 0;-0.000375 -1.06398325290256e-11 -131.246118914422 -82.6228309096625;-0.0003 -1.00587911193696e-11 -128.857332347406 -86.2998428111622;-0.000225 -9.46970886599742e-12 -126.365539200496 -89.9078679387506;-0.00015 -8.87305667224916e-12 -123.772731375006 -93.4440220923452;-7.5e-05 -8.26931149275942e-12 -121.080981521842 -96.9054785244207]  x4=[-0.0006 1.46115216100586e-11 0 0;-0.000525 1.40654778018821e-11 0 0;-0.00045 1.35081902659598e-11 0 0;-0.000375 1.29401044894211e-11 3539.61351587974 -3162.16565183065;-0.0003 1.23616745913438e-11 3627.594285019 -3060.83488284546;-0.000225 1.17733629597382e-11 3712.67521079086 -2957.05732928728;-0.00015 1.11756398819211e-11 3794.78828080505 -2850.91594934455;-7.5e-05 1.05689831685753e-11 3873.86785512978 -2742.49559081239]  x5=0.000588163229675572  V1=ones(3,3)  V2=ones(3,3)  I1=ones(3,3)  I2=ones(3,3)  nHarmo=1  Measurements=None  Decoupling=off  VsMag0=[ 1 1 1]  VrMag0=[ 1 1 1]  VsAngle0=[0 -120 120]  VrAngle0=[0 -120 120]  IsMag0=[ 1 1 1]  IrMag0=[ 1 1 1]  IsAngle0=[0 -120 120]  IrAngle0=[0 -120 120]
      settings: AttributesFormatString=\n  LibrarySourceBlock=sps_lib/Power Grid Elements/Distributed Parameters Line
  LG31-200 MVA : spsSynchronousMachinepuStandardLib/Synchronous Machine pu Standard  PresetModel=No  MechanicalLoad=Mechanical power Pm  ShowDetailedParameters=on  RotorType=Salient-pole  Units=per unit standard parameters  MeasurementBus=off  NominalParameters="[200E6  13800   60 ]"  Reactances1=[ 31 32 33 34 35 36 37 ]  Reactances2=[ 1.305, 0.296, 0.252, 0.474, 0.243, 0.18 ]  dAxisTimeConstants=Short-circuit  qAxisTimeConstants=Open-circuit  TimeConstants1=[]  TimeConstants2=[]  TimeConstants3=[]  TimeConstants4=[]  TimeConstants5=[ 1.01, 0.053, 0.1 ]  TimeConstants6=[]  TimeConstants7=[]  TimeConstants8=[]  StatorResistance=2.8544e-3  Mechanical="[ 3.2  0  32]"  PolePairs=32  InitialConditions=[0 -67.6291 0.902477 0.902477 0.902477 -4.2812 -124.281 115.719 1.45511]  SetSaturation=off  Saturation=[0.6404,0.7127,0.8441,0.9214,0.9956,1.082,1.19,1.316,1.457;0.7,0.7698,0.8872,0.9466,0.9969,1.046,1.1,1.151,1.201]  LoadFlowParameters=[1 180000000 0 0 0]  TsPowergui=0  TsBlock=-1  IterativeModel=Trapezoidal non iterative  IterativeDiscreteModel=Trapezoidal non iterative  BusType=PV  Pref=180000000  Qref=0  Qmin=-Inf  Qmax=Inf  PLF=0  QLF=0
  LG3_2200 MVA : spsSynchronousMachinepuStandardLib/Synchronous Machine pu Standard  PresetModel=No  MechanicalLoad=Mechanical power Pm  ShowDetailedParameters=on  RotorType=Salient-pole  Units=per unit standard parameters  MeasurementBus=off  NominalParameters="[2200E6  13800   60 ]"  Reactances1=[ 31 32 33 34 35 36 37 ]  Reactances2=[ 1.305, 0.296, 0.252, 0.474, 0.243, 0.18 ]  dAxisTimeConstants=Short-circuit  qAxisTimeConstants=Open-circuit  TimeConstants1=[]  TimeConstants2=[]  TimeConstants3=[]  TimeConstants4=[]  TimeConstants5=[ 1.01, 0.053, 0.1 ]  TimeConstants6=[]  TimeConstants7=[]  TimeConstants8=[]  StatorResistance=2.8544e-3  Mechanical="[ 3.2  0  32]"  PolePairs=32  InitialConditions=[0 -70.0065 0.820496 0.820496 0.820496 -4.90643 -124.906 115.094 1.38903]  SetSaturation=off  Saturation=[0.6404,0.7127,0.8441,0.9214,0.9956,1.082,1.19,1.316,1.457;0.7,0.7698,0.8872,0.9466,0.9969,1.046,1.1,1.151,1.201]  LoadFlowParameters=[1 1800000000 0 0 0]  TsPowergui=0  TsBlock=-1  IterativeModel=Trapezoidal non iterative  IterativeDiscreteModel=Trapezoidal non iterative  BusType=PV  Pref=1800000000  Qref=0  Qmin=-Inf  Qmax=Inf  PLF=0  QLF=0
  LG4 660 Mvar : spsThreePhaseSeriesRLCLoadLib/Three-Phase Series RLC Load  LConnTagsString=A|B|C  Configuration=Y (grounded)  NominalVoltage=735e3  Vabc=[1e3 1e3 1e3]  Vabcp=[1e3 1e3 1e3]  NominalFrequency=60  UnbalancedPower=off  ActivePower=2200000  InductivePower=660e6  CapacitivePower=0  Pabc=[10e3 9e3 11e3]  QLabc=[100 90 110]  QCabc=[100 90 110]  Pabcp=[10e3 9e3 11e3]  QLabcp=[100 90 110]  QCabcp=[100 90 110]  Measurements=None  LoadType=constant Z
  LG4-2700 MVA : spsSynchronousMachinepuStandardLib/Synchronous Machine pu Standard  PresetModel=No  MechanicalLoad=Mechanical power Pm  ShowDetailedParameters=on  RotorType=Salient-pole  Units=per unit standard parameters  MeasurementBus=off  NominalParameters="[2700E6  13800   60 ]"  Reactances1=[ 31 32 33 34 35 36 37 ]  Reactances2=[ 1.305, 0.296, 0.252, 0.474, 0.243, 0.18 ]  dAxisTimeConstants=Short-circuit  qAxisTimeConstants=Open-circuit  TimeConstants1=[]  TimeConstants2=[]  TimeConstants3=[]  TimeConstants4=[]  TimeConstants5=[ 1.01, 0.053, 0.1 ]  TimeConstants6=[]  TimeConstants7=[]  TimeConstants8=[]  StatorResistance=2.8544e-3  Mechanical="[ 3.7  0  32]"  PolePairs=32  InitialConditions=[0 -69.506 0.926038 0.926038 0.926038 -2.40174 -122.402 117.598 1.38766]  SetSaturation=off  Saturation=[0.6404,0.7127,0.8441,0.9214,0.9956,1.082,1.19,1.316,1.457;0.7,0.7698,0.8872,0.9466,0.9969,1.046,1.1,1.151,1.201]  LoadFlowParameters=[1 2500000000 0 0 0]  TsPowergui=0  TsBlock=-1  IterativeModel=Trapezoidal non iterative  IterativeDiscreteModel=Trapezoidal non iterative  BusType=PV  Pref=2500000000  Qref=0  Qmin=-Inf  Qmax=Inf  PLF=0  QLF=0
  LG4-LMO 3*118km : spsDistributedParametersLineLib/Distributed Parameters Line  Phases=3  Length=118  Frequency=60  Resistance="[0.01273  0.3864]/3"  Inductance="[0.9337e-3  4.1264e-3]/3"  Capacitance=[12.74e-9 7.751e-9]*3  x1=[-0.000675 -1.12666410897959e-10 442233.573338269 -460179.103702607;-0.0006 -1.13449859524446e-10 455066.323387827 -447492.949543376;-0.000525 -1.1414261806907e-10 467535.300381218 -434449.076367152;-0.00045 -1.14744132751249e-10 479630.536809014 -421057.911246575;-0.000375 -1.15253922729352e-10 491342.363924278 -407330.158874148;-0.0003 -1.15671580485069e-10 502661.419471611 -393276.793005078;-0.000225 -1.15996772149181e-10 513578.655171197 -378909.047685017;-0.00015 -1.16229237768447e-10 524085.343951855 -364238.408269739;-7.5e-05 -1.16368791513408e-10 534173.086927333 -349276.602243925]  x2=[-0.000675 2.56187026116625e-09 410578.900355426 -491671.191825581;-0.0006 2.62559334955073e-09 424314.599421651 -479867.339288629;-0.000525 2.68721757878452e-09 437711.107889329 -467679.888142866;-0.00045 2.74669368740163e-09 450757.716794565 -455118.580850264;-0.000375 2.80397413111085e-09 463443.99687782 -442193.458727678;-0.0003 2.85901312080191e-09 475759.806920902 -428914.853919972;-0.000225 2.91176665914857e-09 487695.3018537 -415293.38114066;-0.00015 2.96219257577943e-09 499240.940624185 -401339.929186666;-7.5e-05 3.01025056098827e-09 510387.493825377 -387065.652233986]  x3=[-0.000675 -2.93018134127574e-11 2132.87241011205 -3249.81810531148;-0.0006 -2.79863109251719e-11 2223.89341215487 -3188.2214934945;-0.000525 -2.66484366088379e-11 2313.13666783073 -3124.07626619704;-0.00045 -2.52892599400134e-11 2400.53083744649 -3057.43370013235;-0.000375 -2.39098674237316e-11 2486.00605944016 -2988.34706834808;-0.0003 -2.25113617252645e-11 2569.49400622707 -2916.87159764062;-0.000225 -2.10948607886696e-11 2650.92793881999 -2843.06442440763;-0.00015 -1.96614969431224e-11 2730.24276017917 -2766.98454897412;-7.5e-05 -1.82124159977499e-11 2807.37506724998 -2688.69278842844]  x4=[-0.000675 3.16220436158573e-11 6469.81651370767 -7978.71819622909;-0.0006 3.03999257525542e-11 6692.79371784066 -7792.62324242294;-0.000525 2.91535066537389e-11 6910.42080507879 -7600.29898482793;-0.00045 2.78837826877682e-11 7122.52380765832 -7401.89916451293;-0.000375 2.65917688525532e-11 7328.93317368428 -7197.58237925867;-0.0003 2.52784979641851e-11 7529.48390266764 -6987.51195677713;-0.000225 2.39450198313184e-11 7724.01567742416 -6771.85582414986;-0.00015 2.25924004159697e-11 7912.37299222956 -6550.78637358963;-7.5e-05 2.12217209814037e-11 8094.40527712834 -6324.48032463275]  x5=0.000667339049054976  V1=ones(3,3)  V2=ones(3,3)  I1=ones(3,3)  I2=ones(3,3)  nHarmo=1  Measurements=None  Decoupling=off  VsMag0=[ 1 1 1]  VrMag0=[ 1 1 1]  VsAngle0=[0 -120 120]  VrAngle0=[0 -120 120]  IsMag0=[ 1 1 1]  IrMag0=[ 1 1 1]  IsAngle0=[0 -120 120]  IrAngle0=[0 -120 120]
      settings: AttributesFormatString=\n  LibrarySourceBlock=sps_lib/Power Grid Elements/Distributed Parameters Line
  LMO 330 Mvar : spsThreePhaseSeriesRLCLoadLib/Three-Phase Series RLC Load  LConnTagsString=A|B|C  Configuration=Y (grounded)  NominalVoltage=735e3  Vabc=[1e3 1e3 1e3]  Vabcp=[1e3 1e3 1e3]  NominalFrequency=60  UnbalancedPower=off  ActivePower=1100000  InductivePower=330e6  CapacitivePower=0  Pabc=[10e3 9e3 11e3]  QLabc=[100 90 110]  QCabc=[100 90 110]  Pabcp=[10e3 9e3 11e3]  QLabcp=[100 90 110]  QCabcp=[100 90 110]  Measurements=None  LoadType=constant Z
  LMO-ALB 3*218km : spsDistributedParametersLineLib/Distributed Parameters Line  Phases=3  Length=218  Frequency=60  Resistance="[0.01273  0.3864]/3"  Inductance="[0.9337e-3  4.1264e-3]/3"  Capacitance=[12.74e-9 7.751e-9]*3  x1=[-0.001275 1.98297226721028e-09 0 0;-0.0012 2.06152035433679e-09 0 0;-0.001125 2.13842049363436e-09 0 0;-0.00105 2.21361121230825e-09 0 0;-0.000975 2.28703240404841e-09 0 0;-0.0009 2.35862537707754e-09 0 0;-0.000825 2.42833290106841e-09 382134.113224462 -514090.671982308;-0.00075 2.49609925289291e-09 396514.990798325 -503082.009934609;-0.000675 2.56187026116625e-09 410578.900355426 -491671.191825581;-0.0006 2.62559334955073e-09 424314.599421651 -479867.339288629;-0.000525 2.68721757878452e-09 437711.107889329 -467679.888142866;-0.00045 2.74669368740163e-09 450757.716794565 -455118.580850264;-0.000375 2.80397413111085e-09 463443.99687782 -442193.458727678;-0.0003 2.85901312080191e-09 475759.806920902 -428914.853919972;-0.000225 2.91176665914857e-09 487695.3018537 -415293.38114066;-0.00015 2.96219257577943e-09 499240.940624185 -401339.929186666;-7.5e-05 3.01025056098827e-09 510387.493825377 -387065.652233986]  x2=[-0.001275 5.96918622325256e-09 0 0;-0.0012 6.21440045910552e-09 0 0;-0.001125 6.45464699831498e-09 0 0;-0.00105 6.6897337914734e-09 0 0;-0.000975 6.91947291379528e-09 0 0;-0.0009 7.14368071534135e-09 0 0;-0.000825 7.36217796782556e-09 256872.501303786 -581628.877217016;-0.00075 7.57479000788739e-09 273212.791419988 -574134.441892282;-0.000675 7.78134687671509e-09 289334.679411025 -566181.05227925;-0.0006 7.98168345590814e-09 305225.27768631 -557775.066195887;-0.000525 8.17563959947039e-09 320871.883544716 -548923.203258852;-0.00045 8.36306026182831e-09 336261.98932892 -539632.539511939;-0.000375 8.54379562177203e-09 351383.292423836 -529910.501769594;-0.0003 8.71770120222016e-09 366223.705091133 -519764.861680037;-0.000225 8.88463798571254e-09 380771.364131991 -509203.729512722;-0.00015 9.04447252553867e-09 395014.640370359 -498235.547675114;-7.5e-05 9.19707705241294e-09 408942.147949142 -486869.083963953]  x3=[-0.001275 -3.66856481718819e-11 0 0;-0.0012 -3.50495050158731e-11 0 0;-0.001125 -3.338534382183e-11 0 0;-0.00105 -3.16944948947486e-11 0 0;-0.000975 -2.99783098733904e-11 0 0;-0.0009 -2.82381606498029e-11 0 0;-0.000825 -2.64754382726503e-11 558.937753072927 -1417.04584856712;-0.00075 -2.46915518352304e-11 598.774931611999 -1400.67750101635;-0.000675 -2.28879273490668e-11 638.133458632303 -1383.18947330235;-0.0006 -2.10660066039773e-11 676.981871529547 -1364.59574508691;-0.000525 -1.92272460155294e-11 715.289115476859 -1344.91117991185;-0.00045 -1.73731154608034e-11 753.02456824955 -1324.15151331741;-0.000375 -1.55050971033955e-11 790.158064704044 -1302.33334026342;-0.0003 -1.36246842085992e-11 826.659920891438 -1279.47410186358;-0.000225 -1.17333799497112e-11 862.500957786392 -1255.59207144333;-0.00015 -9.8326962064181e-12 897.652524612399 -1230.70633993237;-7.5e-05 -7.9241523562229e-12 932.086521744775 -1204.83680060371]  x4=[-0.001275 5.61550290783206e-11 0 0;-0.0012 5.59750627675318e-11 0 0;-0.001125 5.57503508480138e-11 0 0;-0.00105 5.54810729510369e-11 0 0;-0.000975 5.51674443332318e-11 0 0;-0.0009 5.48097157045169e-11 0 0;-0.000825 5.44081730276846e-11 4744.0729156647 -11636.8846137319;-0.00075 5.3963137289807e-11 5071.15764281527 -11498.1156070747;-0.000675 5.34749642456435e-11 5394.18856413749 -11350.1551827283;-0.0006 5.29440441332565e-11 5712.90745365538 -11193.1216179921;-0.000525 5.23708013620604e-11 6027.05953236524 -11027.1404430949;-0.00045 5.17556941735556e-11 6336.39367190203 -10852.3443408485;-0.000375 5.10992142750171e-11 6640.66259528758 -10668.8730405824;-0.0003 5.04018864464314e-11 6939.6230746 -10476.8732064468;-0.000225 4.96642681209951e-11 7233.03612540638 -10276.4983201716;-0.00015 4.88869489395117e-11 7520.66719780327 -10067.908558375;-7.5e-05 4.80705502790414e-11 7802.2863639123 -9851.2706645209]  x5=0.00123288061605072  V1=ones(3,3)  V2=ones(3,3)  I1=ones(3,3)  I2=ones(3,3)  nHarmo=1  Measurements=None  Decoupling=off  VsMag0=[ 1 1 1]  VrMag0=[ 1 1 1]  VsAngle0=[0 -120 120]  VrAngle0=[0 -120 120]  IsMag0=[ 1 1 1]  IrMag0=[ 1 1 1]  IsAngle0=[0 -120 120]  IrAngle0=[0 -120 120]
      settings: AttributesFormatString=\n  LibrarySourceBlock=sps_lib/Power Grid Elements/Distributed Parameters Line
  LMO7 : spsThreePhaseVIMeasurementLib/Three-Phase V-I Measurement  VoltageMeasurement=no  SetLabelV=on  LabelV=Vabc_LMO7  Vpu=on  VpuLL=off  CurrentMeasurement=no  SetLabelI=off  LabelI=A1  Ipu=off  Pbase=100e6  Vbase=735e3  OutputType=Magnitude  PhasorSimulation=off  PSBequivalent=0
  LVD 990 Mvar : spsThreePhaseSeriesRLCLoadLib/Three-Phase Series RLC Load  LConnTagsString=A|B|C  Configuration=Y (grounded)  NominalVoltage=735e3  Vabc=[1e3 1e3 1e3]  Vabcp=[1e3 1e3 1e3]  NominalFrequency=60  UnbalancedPower=off  ActivePower=3300000  InductivePower=990e6  CapacitivePower=0  Pabc=[10e3 9e3 11e3]  QLabc=[100 90 110]  QCabc=[100 90 110]  Pabcp=[10e3 9e3 11e3]  QLabcp=[100 90 110]  QCabcp=[100 90 110]  Measurements=None  LoadType=constant Z
  LVD-MTL 3*260km : spsDistributedParametersLineLib/Distributed Parameters Line  Phases=3  Length=260  Frequency=60  Resistance="[0.01273  0.3864]/3"  Inductance="[0.9337e-3  4.1264e-3]/3"  Capacitance=[12.74e-9 7.751e-9]*3  x1=[-0.0015 1.72989899597864e-08 -60766.0885086435 -643710.808029355;-0.001425 1.81491216960882e-08 -42543.7444111707 -645171.399881573;-0.00135 1.89847453021969e-08 -24287.3914953567 -646116.251588179;-0.001275 1.98051927933875e-08 -6011.62361039087 -646544.607849175;-0.0012 2.06098083164886e-08 12268.9498745082 -646456.126243122;-0.001125 2.13979486741622e-08 30539.7157485987 -645850.877500859;-0.00105 2.21689838390653e-08 48786.0686411932 -644729.345448972;-0.000975 2.29222974574842e-08 66993.4226969678 -643092.426623024;-0.0009 2.36572873420385e-08 85147.2232356722 -640941.429550877;-0.000825 2.43733659530602e-08 103232.958386918 -638278.073706679;-0.00075 2.50699608682641e-08 121236.170690747 -635104.488136342;-0.000675 2.57465152403331e-08 139142.468654701 -631423.209755614;-0.0006 2.64024882420539e-08 156937.538258164 -627237.181322107;-0.000525 2.70373554986456e-08 174607.154394768 -622549.749082901;-0.00045 2.76506095069372e-08 192137.192243728 -617364.660099608;-0.000375 2.82417600410573e-08 209513.638561005 -611686.059253028;-0.0003 2.88103345443141e-08 226722.602881284 -605518.485929792;-0.000225 2.93558785069491e-08 243750.328621791 -598866.870393647;-0.00015 2.98779558294656e-08 260583.204079103 -591736.52984428;-7.5e-05 3.03761491712401e-08 277207.773310131 -584133.164166828]  x2=[-0.0015 2.83327978437215e-08 -284434.156182434 -570661.101567503;-0.001425 2.95898889264445e-08 -268187.556421239 -578474.126624351;-0.00135 3.08233263047001e-08 -251726.571630847 -585824.728315327;-0.001275 3.20321239875206e-08 -235064.36047064 -592707.030681907;-0.0012 3.32153156805333e-08 -218214.242457277 -599115.532116881;-0.001125 3.43719555584024e-08 -201189.687317284 -605045.109762256;-0.00105 3.55011190209066e-08 -184004.304219555 -610491.023604388;-0.000975 3.66019034320509e-08 -166671.830896394 -615448.920263076;-0.0009 3.76734288416195e-08 -149206.122661778 -619914.83647159;-0.000825 3.87148386885949e-08 -131621.141335636 -623885.202244844;-0.00075 3.97253004858795e-08 -113930.944082982 -627356.843733187;-0.000675 4.07040064857732e-08 -96149.6721768303 -630326.985759531;-0.0006 4.16501743256744e-08 -78291.5396938793 -632793.254037786;-0.000525 4.25630476534886e-08 -60370.8221519978 -634753.677070824;-0.00045 4.34418967322451e-08 -42401.8450985925 -636206.687726468;-0.000375 4.42860190234372e-08 -24398.9726589854 -637151.124490233;-0.0003 4.50947397486207e-08 -6376.59605395151 -637586.23239382;-0.000225 4.58674124288219e-08 11650.8779044027 -637511.663618627;-0.00015 4.66034194013224e-08 29669.0383292246 -636927.477773793;-7.5e-05 4.73021723134097e-08 47663.4817787576 -635834.141848544]  x3=[-0.0015 -5.16611824434392e-11 283.845435905075 550.505795112931;-0.001425 -4.5139929097673e-11 268.169144865239 558.310803130099;-0.00135 -3.85825915832502e-11 252.278483514124 565.669506033687;-0.001275 -3.19944117354492e-11 236.186154603277 572.576021389185;-0.0012 -2.53806560444378e-11 219.90502209421 579.024828233891;-0.001125 -1.87466114453216e-11 203.44810087514 585.010771490284;-0.00105 -1.20975810918487e-11 186.828546357091 590.529066086913;-0.000975 -5.43888011715023e-12 170.059643957657 595.57530078351;-0.0009 1.22416861509626e-12 153.154798480843 600.145441697268;-0.000825 7.88623876568224e-12 136.127523401471 604.235835527466;-0.00075 1.45420047776624e-11 118.991430062712 607.843212475862;-0.000675 2.11861461335235e-11 101.760216795391 610.964688860518;-0.0006 2.78133516083243e-11 84.4476579677472 613.597769420972;-0.000525 3.4418323515408e-11 67.0675929744166 615.740349312911;-0.00045 4.09957819412915e-11 49.6339151734308 617.390715790753;-0.000375 4.75404689663476e-11 32.1605607800797 618.547549576787;-0.0003 5.40471528679056e-11 14.6614977265141 619.209925915784;-0.000225 6.05106323024101e-11 -2.84928550400558 619.377315314233;-0.00015 6.69257404632959e-11 -20.3577910592889 619.049583963611;-7.5e-05 7.32873492112534e-11 -37.8500229078841 618.226993847344]  x4=[-0.0015 1.38095018815547e-10 -6356.55576531306 -13234.8737869081;-0.001425 1.40801650501511e-10 -5979.85814727543 -13409.2877766846;-0.00135 1.43395727502402e-10 -5598.38032212976 -13572.9825869815;-0.001275 1.45875176152756e-10 -5212.42723741267 -13725.8273626718;-0.0012 1.48238014419259e-10 -4822.30741811481 -13867.6999219807;-0.001125 1.50482353485152e-10 -4428.33272005068 -13998.4868541549;-0.00105 1.52606399260127e-10 -4030.8180805659 -14118.0836101219;-0.000975 1.54608453814489e-10 -3630.08126678111 -14226.3945860648;-0.0009 1.5648691673646e-10 -3226.44262157376 -14323.3331998469;-0.000825 1.58240286411523e-10 -2820.22480750095 -14408.8219602233;-0.00075 1.59867161222786e-10 -2411.75254886791 -14482.792528787;-0.000675 1.61366240671416e-10 -2001.35237214836 -14545.1857745974;-0.0006 1.62736326416241e-10 -1589.35234496422 -14595.9518214484;-0.000525 1.63976323231677e-10 -1176.08181383344 -14635.0500877389;-0.00045 1.65085239883244e-10 -761.871140895323 -14662.4493189131;-0.000375 1.66062189919937e-10 -347.051439824198 -14678.1276124446;-0.0003 1.66906392382845e-10 68.0456888578574 -14682.0724353457;-0.000225 1.67617172429436e-10 483.088422857373 -14674.2806341852;-0.00015 1.68193961873015e-10 897.744983363158 -14654.7584376098;-7.5e-05 1.68636299636927e-10 1311.6839002652 -14623.5214513647]  x5=0.00147040807418893  V1=ones(3,3)  V2=ones(3,3)  I1=ones(3,3)  I2=ones(3,3)  nHarmo=1  Measurements=None  Decoupling=off  VsMag0=[ 1 1 1]  VrMag0=[ 1 1 1]  VsAngle0=[0 -120 120]  VrAngle0=[0 -120 120]  IsMag0=[ 1 1 1]  IrMag0=[ 1 1 1]  IsAngle0=[0 -120 120]  IrAngle0=[0 -120 120]
      settings: AttributesFormatString=\n  LibrarySourceBlock=sps_lib/Power Grid Elements/Distributed Parameters Line
  LVD7 : spsThreePhaseVIMeasurementLib/Three-Phase V-I Measurement  VoltageMeasurement=no  SetLabelV=on  LabelV=Vabc_LVD7  Vpu=on  VpuLL=off  CurrentMeasurement=no  SetLabelI=off  LabelI=A1  Ipu=off  Pbase=100e6  Vbase=735e3  OutputType=Magnitude  PhasorSimulation=off  PSBequivalent=0
  Load Flow Bus1 : spsLoadFlowBusLib/Load Flow Bus  LConnTagsString=a  Phases=single  Connectors=on one side  ID=LG31_13.8  Vbase=13.8e3  Vref=1  Vangle=0  VLF=1  VLFb=1  VLFc=1  angleLF=-0.0351  angleLFb=0  angleLFc=0
      settings: AttributesFormatString=%<ID>\n%<Vbase>V\n%<VLF>pu\n%<angleLF>deg.
  Load Flow Bus10 : spsLoadFlowBusLib/Load Flow Bus  LConnTagsString=a  Phases=single  Connectors=on one side  ID=LVD7  Vbase=735e3  Vref=1  Vangle=0  VLF=1.05  VLFb=1  VLFc=1  angleLF=-12.02  angleLFb=0  angleLFc=0
      settings: AttributesFormatString=%<ID>\n%<Vbase>V\n%<VLF>pu\n%<angleLF>deg.
  Load Flow Bus11 : spsLoadFlowBusLib/Load Flow Bus  LConnTagsString=a  Phases=single  Connectors=on one side  ID=CHM7  Vbase=735e3  Vref=1  Vangle=0  VLF=1.047  VLFb=1  VLFc=1  angleLF=-4.064  angleLFb=0  angleLFc=0
      settings: AttributesFormatString=%<ID>\n%<Vbase>V\n%<VLF>pu\n%<angleLF>deg.
  Load Flow Bus12 : spsLoadFlowBusLib/Load Flow Bus  LConnTagsString=a  Phases=single  Connectors=on one side  ID=LG47  Vbase=735e3  Vref=1  Vangle=0  VLF=1.004  VLFb=1  VLFc=1  angleLF=20.71  angleLFb=0  angleLFc=0
      settings: AttributesFormatString=%<ID>\n%<Vbase>V\n%<VLF>pu\n%<angleLF>deg.
  Load Flow Bus2 : spsLoadFlowBusLib/Load Flow Bus  LConnTagsString=a  Phases=single  Connectors=on one side  ID=LG3_13.8  Vbase=13.8e3  Vref=1  Vangle=0  VLF=1  VLFb=1  VLFc=1  angleLF=-0.6025  angleLFb=0  angleLFc=0
      settings: AttributesFormatString=%<ID>\n%<Vbase>V\n%<VLF>pu\n%<angleLF>deg.
  Load Flow Bus3 : spsLoadFlowBusLib/Load Flow Bus  LConnTagsString=a  Phases=single  Connectors=on one side  ID=LG4_13.8  Vbase=13.8e3  Vref=1  Vangle=0  VLF=1  VLFb=1  VLFc=1  angleLF=-3.293  angleLFb=0  angleLFc=0
      settings: AttributesFormatString=%<ID>\n%<Vbase>V\n%<VLF>pu\n%<angleLF>deg.
  Load Flow Bus4 : spsLoadFlowBusLib/Load Flow Bus  LConnTagsString=a  Phases=single  Connectors=on one side  ID=LG2_13.8  Vbase=13.8e3  Vref=1  Vangle=0  VLF=1  VLFb=1  VLFc=1  angleLF=0  angleLFb=0  angleLFc=0
      settings: AttributesFormatString=%<ID>\n%<Vbase>V\n%<VLF>pu\n%<angleLF>deg.
  Load Flow Bus5 : spsLoadFlowBusLib/Load Flow Bus  LConnTagsString=a  Phases=single  Connectors=on one side  ID=LG27  Vbase=735e3  Vref=1  Vangle=0  VLF=1  VLFb=1  VLFc=1  angleLF=23.57  angleLFb=0  angleLFc=0
      settings: AttributesFormatString=%<ID>\n%<Vbase>V\n%<VLF>pu\n%<angleLF>deg.
  Load Flow Bus6 : spsLoadFlowBusLib/Load Flow Bus  LConnTagsString=a  Phases=single  Connectors=on one side  ID=LG37  Vbase=735e3  Vref=1  Vangle=0  VLF=0.994  VLFb=1  VLFc=1  angleLF=24.1  angleLFb=0  angleLFc=0
      settings: AttributesFormatString=%<ID>\n%<Vbase>V\n%<VLF>pu\n%<angleLF>deg.
  Load Flow Bus7 : spsLoadFlowBusLib/Load Flow Bus  LConnTagsString=a  Phases=single  Connectors=on one side  ID=LMO7  Vbase=735e3  Vref=1  Vangle=0  VLF=1.016  VLFb=1  VLFc=1  angleLF=17.31  angleLFb=0  angleLFc=0
      settings: AttributesFormatString=%<ID>\n%<Vbase>V\n%<VLF>pu\n%<angleLF>deg.
  Load Flow Bus8 : spsLoadFlowBusLib/Load Flow Bus  LConnTagsString=a  Phases=single  Connectors=on one side  ID=NEM_ALB7  Vbase=735e3  Vref=1  Vangle=0  VLF=1.028  VLFb=1  VLFc=1  angleLF=8.928  angleLFb=0  angleLFc=0
      settings: AttributesFormatString=%<ID>\n%<Vbase>V\n%<VLF>pu\n%<angleLF>deg.
  Load Flow Bus9 : spsLoadFlowBusLib/Load Flow Bus  LConnTagsString=a  Phases=single  Connectors=on one side  ID=ABI_CHB7  Vbase=735e3  Vref=1  Vangle=0  VLF=1.046  VLFb=1  VLFc=1  angleLF=0.1334  angleLFb=0  angleLFc=0
      settings: AttributesFormatString=%<ID>\n%<Vbase>V\n%<VLF>pu\n%<angleLF>deg.
  NEM-ABI 6*236 : spsDistributedParametersLineLib/Distributed Parameters Line  Phases=3  Length=236  Frequency=60  Resistance="[0.01273  0.3864]/6"  Inductance="[0.9337e-3  4.1264e-3]/6"  Capacitance=[12.74e-9 7.751e-9]*6  x1=[-0.00135 5.63061764000322e-09 0 0;-0.001275 5.89525893642959e-09 0 0;-0.0012 6.15518765306266e-09 0 0;-0.001125 6.41019600686341e-09 0 0;-0.00105 6.66008014805556e-09 0 0;-0.000975 6.90464032307999e-09 0 0;-0.0009 7.1436810342747e-09 0 0;-0.000825 7.37701119615259e-09 284967.297433621 -571339.995920179;-0.00075 7.60444428815233e-09 301005.484998393 -563055.415941782;-0.000675 7.82579850374002e-09 316803.053383995 -554320.738078918;-0.0006 8.04089689574256e-09 332347.374255972 -545142.944699425;-0.000525 8.24956751779649e-09 347626.021722054 -535529.372390906;-0.00045 8.4516435617993e-09 362626.782265227 -525487.706095972;-0.000375 8.6469634912533e-09 377337.664507034 -515025.972969016;-0.0003 8.83537117039537e-09 391746.908793294 -504152.535959431;-0.000225 9.01671598900953e-09 405842.996594592 -492876.087126392;-0.00015 9.19085298282246e-09 419614.65971402 -481205.640690561;-7.5e-05 9.35764294938569e-09 433050.889294791 -469150.525828256]  x2=[-0.00135 1.06661708509858e-08 0 0;-0.001275 1.10873744772551e-08 0 0;-0.0012 1.14997150260099e-08 0 0;-0.001125 1.19028628785245e-08 0 0;-0.00105 1.22964957645738e-08 0 0;-0.000975 1.26802990200517e-08 0 0;-0.0009 1.3053965838508e-08 0 0;-0.000825 1.34171975164053e-08 124240.179514877 -633974.103134436;-0.00075 1.37697036918981e-08 142113.319168641 -630208.35351111;-0.000675 1.41112025769431e-08 159872.855609468 -625938.8249725;-0.0006 1.44414211825567e-08 177504.592135658 -621168.930514391;-0.000525 1.47600955370381e-08 194994.434206806 -615902.483117432;-0.00045 1.50669708969843e-08 212328.400710763 -610143.692699094;-0.000375 1.53618019509278e-08 229492.635139926 -603897.162748323;-0.0003 1.56443530154352e-08 246473.416667914 -597167.886645588;-0.000225 1.59143982235086e-08 263257.171117786 -589961.243671243;-0.00015 1.61717217051407e-08 279830.481813037 -582282.994705417;-7.5e-05 1.64161177598773e-08 296180.100302677 -574139.277622852]  x3=[-0.00135 -4.21134501749124e-11 0 0;-0.001275 -3.71124663051307e-11 0 0;-0.0012 -3.20818152976245e-11 0 0;-0.001125 -2.70255185778376e-11 0 0;-0.00105 -2.19476180720038e-11 0 0;-0.000975 -1.68521729760931e-11 0 0;-0.0009 -1.17432565109523e-11 0 0;-0.000825 -6.62495266623439e-12 -663.961228469135 -1977.20263991353;-0.00075 -1.5013529357203e-12 -607.798395730439 -1995.1816636065;-0.000675 3.62344695335915e-12 -551.149698253822 -2011.56576960488;-0.0006 8.74535031438466e-12 -494.060420141295 -2026.34186070503;-0.000525 1.38602627761772e-11 -436.576197688285 -2039.4981251258;-0.00045 1.89640955559756e-11 -378.742982902682 -2051.02404595071;-0.000375 2.4052768727947e-11 -320.607006771509 -2060.91040953501;-0.0003 2.91222144846169e-11 -262.214742304575 -2069.14931287091;-0.000225 3.41683803886127e-11 -203.612867384663 -2075.73416990515;-0.00015 3.91872326121195e-11 -144.848227453944 -2080.65971680377;-7.5e-05 4.4174759161461e-11 -85.967798066451 -2083.92201615993]  x4=[-0.00135 1.16942912524546e-10 0 0;-0.001275 1.1791104785875e-10 0 0;-0.0012 1.18784926905395e-10 0 0;-0.001125 1.19563851098942e-10 0 0;-0.00105 1.20247197779309e-10 0 0;-0.000975 1.20834420689614e-10 0 0;-0.0009 1.2132505041285e-10 0 0;-0.000825 1.2171869474712e-10 5549.38040349503 -25908.0748550802;-0.00075 1.22015039019169e-10 6279.5967194177 -25740.83578365;-0.000675 1.22213846335918e-10 7004.79322180392 -25553.0198819424;-0.0006 1.2231495777384e-10 7724.39019966556 -25344.7772871155;-0.000525 1.22318292506e-10 8437.81241818872 -25116.2744651133;-0.00045 1.22223847866664e-10 9144.48957856764 -24867.6940775956;-0.000375 1.2203169935343e-10 9843.85677389284 -24599.2348359208;-0.0003 1.21742000566881e-10 10535.354940729 -24311.1113422991;-0.000225 1.21354983087793e-10 11218.431306022 -24003.5539182428;-0.00015 1.20870956292019e-10 11892.5398289766 -23676.8084204509;-7.5e-05 1.20290307103172e-10 12557.1416375539 -23331.1360442751]  x5=0.00133467809810995  V1=ones(3,3)  V2=ones(3,3)  I1=ones(3,3)  I2=ones(3,3)  nHarmo=1  Measurements=None  Decoupling=off  VsMag0=[ 1 1 1]  VrMag0=[ 1 1 1]  VsAngle0=[0 -120 120]  VrAngle0=[0 -120 120]  IsMag0=[ 1 1 1]  IrMag0=[ 1 1 1]  IsAngle0=[0 -120 120]  IrAngle0=[0 -120 120]
      settings: AttributesFormatString=\n  LibrarySourceBlock=sps_lib/Power Grid Elements/Distributed Parameters Line
  NEM-ALB 1980 Mvar : spsThreePhaseSeriesRLCLoadLib/Three-Phase Series RLC Load  LConnTagsString=A|B|C  Configuration=Y (grounded)  NominalVoltage=735e3  Vabc=[1e3 1e3 1e3]  Vabcp=[1e3 1e3 1e3]  NominalFrequency=60  UnbalancedPower=off  ActivePower=6600000  InductivePower=1980e6  CapacitivePower=0  Pabc=[10e3 9e3 11e3]  QLabc=[100 90 110]  QCabc=[100 90 110]  Pabcp=[10e3 9e3 11e3]  QLabcp=[100 90 110]  QCabcp=[100 90 110]  Measurements=None  LoadType=constant Z
  NEM-ALB7 : spsThreePhaseVIMeasurementLib/Three-Phase V-I Measurement  VoltageMeasurement=no  SetLabelV=on  LabelV=Vabc_NEM7  Vpu=on  VpuLL=off  CurrentMeasurement=no  SetLabelI=off  LabelI=A1  Ipu=off  Pbase=100e6  Vbase=735e3  OutputType=Magnitude  PhasorSimulation=off  PSBequivalent=0
  Regulators1 : Subsystem
  Regulators2 : Subsystem
  Regulators3 : Subsystem
  Regulators4 : Subsystem
  MTLa : PMIOPort  Side=Right
  MTLb : PMIOPort  Port=2  Side=Right
  MTLc : PMIOPort  Port=3  Side=Right
  CHM7a : PMIOPort  Port=4  Side=Right
  CHM7b : PMIOPort  Port=5  Side=Right
  CHM7c : PMIOPort  Port=6  Side=Right
  wires:
  Regulators2/1(Pm) -> LG3_2200 MVA/1
  Regulators4/2(Vf) -> LG4-2700 MVA/2
  Regulators4/1(Pm) -> LG4-2700 MVA/1
  Regulators3/2(Vf) -> LG31-200 MVA/2
  Regulators3/1(Pm) -> LG31-200 MVA/1
  Regulators2/2(Vf) -> LG3_2200 MVA/2
  LG3_2200 MVA/1 -> Regulators2/1(m)
  Regulators1/1(Pm) -> LG2_5500 MVA/1
  Regulators1/2(Vf) -> LG2_5500 MVA/2
  LG2_5500 MVA/1 -> Regulators1/1(m)
  LG31-200 MVA/1 -> Regulators3/1(m)
  LG4-2700 MVA/1 -> Regulators4/1(m)
  connections:
  LG2-NENI 3*279km/RConn1 -- "Cs NEM "/LConn1
  LG2-NENI 3*279km/RConn2 -- "Cs NEM "/LConn2
  LG2-NENI 3*279km/RConn3 -- "Cs NEM "/LConn3
  CHB-CHM 3*195km/RConn1 -- "Cs  CHMN "/LConn1
  CHB-CHM 3*195km/RConn2 -- "Cs  CHMN "/LConn2
  CHB-CHM 3*195km/RConn3 -- "Cs  CHMN "/LConn3
  Load Flow Bus2/LConn1 -- 2200 MVA 13.8 kV/735 kV/LConn1 -- LG3_2200 MVA/RConn1 -- 110 MW/LConn1
  2200 MVA 13.8 kV/735 kV/LConn2 -- LG3_2200 MVA/RConn2 -- 110 MW/LConn2
  2200 MVA 13.8 kV/735 kV/LConn3 -- LG3_2200 MVA/RConn3 -- 110 MW/LConn3
  Load Flow Bus1/LConn1 -- 200 MVA 13.8 kV/735 kV/LConn1 -- LG31-200 MVA/RConn1 -- 10 MW/LConn1
  200 MVA 13.8 kV/735 kV/LConn2 -- LG31-200 MVA/RConn2 -- 10 MW/LConn2
  200 MVA 13.8 kV/735 kV/LConn3 -- LG31-200 MVA/RConn3 -- 10 MW/LConn3
  Load Flow Bus6/LConn1 -- 2200 MVA 13.8 kV/735 kV/RConn1 -- 200 MVA 13.8 kV/735 kV/RConn1 -- LG3-LMO 104km/LConn1 -- LG3 660 Mvar/LConn1 -- LG2-LG3 155km/RConn1
  2200 MVA 13.8 kV/735 kV/RConn2 -- LG3 660 Mvar/LConn2 -- LG2-LG3 155km/RConn2 -- 200 MVA 13.8 kV/735 kV/RConn2 -- LG3-LMO 104km/LConn2
  LG3-LMO 104km/RConn1 -- LMO7/RConn1 -- LG4-LMO 3*118km/RConn1 -- LMO 330 Mvar/LConn1
  LG3-LMO 104km/RConn2 -- LMO7/RConn2 -- LG4-LMO 3*118km/RConn2 -- LMO 330 Mvar/LConn2
  LG3-LMO 104km/RConn3 -- LMO7/RConn3 -- LG4-LMO 3*118km/RConn3 -- LMO 330 Mvar/LConn3
  LG4-LMO 3*118km/LConn1 -- LG4 660 Mvar/LConn1 -- 2700 MVA 13.8 kV/735 kV/RConn1 -- Load Flow Bus12/LConn1
  LG4-LMO 3*118km/LConn2 -- 2700 MVA 13.8 kV/735 kV/RConn2 -- LG4 660 Mvar/LConn2
  LG4 660 Mvar/LConn3 -- 2700 MVA 13.8 kV/735 kV/RConn3 -- LG4-LMO 3*118km/LConn3
  Load Flow Bus3/LConn1 -- LG4-2700 MVA/RConn1 -- 2700 MVA 13.8 kV/735 kV/LConn1 -- 135 MW/LConn1
  LG4-2700 MVA/RConn2 -- 2700 MVA 13.8 kV/735 kV/LConn2 -- 135 MW/LConn2
  LG4-2700 MVA/RConn3 -- 2700 MVA 13.8 kV/735 kV/LConn3 -- 135 MW/LConn3
  Load Flow Bus4/LConn1 -- 5500 MVA 13.8 kV/735 kV/LConn1 -- LG2_5500 MVA/RConn1 -- 275 MW/LConn1
  5500 MVA 13.8 kV/735 kV/LConn2 -- LG2_5500 MVA/RConn2 -- 275 MW/LConn2
  LG2_5500 MVA/RConn3 -- 5500 MVA 13.8 kV/735 kV/LConn3 -- 275 MW/LConn3
  5500 MVA 13.8 kV/735 kV/RConn1 -- LG2-NENI 3*279km/LConn1 -- LG2-LG3 155km/LConn1 -- LG2 660 Mvar/LConn1 -- Load Flow Bus5/LConn1
  LG2-LG3 155km/LConn2 -- 5500 MVA 13.8 kV/735 kV/RConn2 -- LG2-NENI 3*279km/LConn2 -- LG2 660 Mvar/LConn2
  LG2-LG3 155km/LConn3 -- 5500 MVA 13.8 kV/735 kV/RConn3 -- LG2-NENI 3*279km/LConn3 -- LG2 660 Mvar/LConn3
  "Cs NEM "/RConn1 -- NEM-ALB7/LConn1 -- Cs ALB/RConn1
  "Cs NEM "/RConn2 -- NEM-ALB7/LConn2 -- Cs ALB/RConn2
  "Cs NEM "/RConn3 -- NEM-ALB7/LConn3 -- Cs ALB/RConn3
  LMO7/LConn1 -- LMO-ALB 3*218km/LConn1
  LMO7/LConn2 -- LMO-ALB 3*218km/LConn2
  Load Flow Bus7/LConn1 -- LMO7/LConn3 -- LMO-ALB 3*218km/LConn3
  Cs ALB/LConn1 -- LMO-ALB 3*218km/RConn1
  Cs ALB/LConn2 -- LMO-ALB 3*218km/RConn2
  Cs ALB/LConn3 -- LMO-ALB 3*218km/RConn3
  200 MVA 13.8 kV/735 kV/RConn3 -- LG3-LMO 104km/LConn3 -- LG3 660 Mvar/LConn3 -- LG2-LG3 155km/RConn3 -- 2200 MVA 13.8 kV/735 kV/RConn3
  Load Flow Bus8/LConn1 -- NEM-ABI 6*236/LConn1 -- NEM-ALB7/RConn1 -- NEM-ALB 1980 Mvar/LConn1
  NEM-ALB 1980 Mvar/LConn2 -- NEM-ALB7/RConn2 -- NEM-ABI 6*236/LConn2
  NEM-ALB 1980 Mvar/LConn3 -- NEM-ALB7/RConn3 -- NEM-ABI 6*236/LConn3
  NEM-ABI 6*236/RConn1 -- "Cs ABI+CHB "/LConn1
  NEM-ABI 6*236/RConn2 -- "Cs ABI+CHB "/LConn2
  NEM-ABI 6*236/RConn3 -- "Cs ABI+CHB "/LConn3
  "Cs ABI+CHB "/RConn1 -- ABI-CHB7/LConn1
  "Cs ABI+CHB "/RConn2 -- ABI-CHB7/LConn2
  "Cs ABI+CHB "/RConn3 -- ABI-CHB7/LConn3
  Load Flow Bus9/LConn1 -- ABI+CHB 1320 Mvar/LConn1 -- CHB-CHM 3*195km/LConn1 -- ABI-CHB 3*271km/LConn1 -- ABI-CHB7/RConn1
  ABI-CHB 3*271km/LConn2 -- ABI-CHB7/RConn2 -- ABI+CHB 1320 Mvar/LConn2 -- CHB-CHM 3*195km/LConn2
  ABI-CHB 3*271km/LConn3 -- ABI-CHB7/RConn3 -- ABI+CHB 1320 Mvar/LConn3 -- CHB-CHM 3*195km/LConn3
  ABI-CHB 3*271km/RConn1 -- "Cs LVDN "/LConn1
  ABI-CHB 3*271km/RConn2 -- "Cs LVDN "/LConn2
  ABI-CHB 3*271km/RConn3 -- "Cs LVDN "/LConn3
  "Cs LVDN "/RConn1 -- LVD7/LConn1
  "Cs LVDN "/RConn2 -- LVD7/LConn2
  "Cs LVDN "/RConn3 -- LVD7/LConn3
  "Cs LVDS "/LConn1 -- LVD 990 Mvar/LConn1 -- Load Flow Bus10/LConn1 -- LVD7/RConn1
  "Cs LVDS "/LConn2 -- LVD7/RConn2 -- LVD 990 Mvar/LConn2
  "Cs LVDS "/LConn3 -- LVD7/RConn3 -- LVD 990 Mvar/LConn3
  "Cs LVDS "/RConn1 -- LVD-MTL 3*260km/LConn1
  "Cs LVDS "/RConn2 -- LVD-MTL 3*260km/LConn2
  "Cs LVDS "/RConn3 -- LVD-MTL 3*260km/LConn3
  MTLa/RConn1 -- LVD-MTL 3*260km/RConn1
  MTLb/RConn1 -- LVD-MTL 3*260km/RConn2
  MTLc/RConn1 -- LVD-MTL 3*260km/RConn3
  "Cs  CHMN "/RConn1 -- CHM7/LConn1
  "Cs  CHMN "/RConn2 -- CHM7/LConn2
  "Cs  CHMN "/RConn3 -- CHM7/LConn3
  CHM 1320Mvar/LConn2 -- CHM7/RConn2 -- CHM7b/RConn1
  Load Flow Bus11/LConn1 -- CHM 1320Mvar/LConn3 -- CHM7c/RConn1 -- CHM7/RConn3
  CHM7a/RConn1 -- CHM 1320Mvar/LConn1 -- CHM7/RConn1
